simulink model "DesacopleDeTensiones"  (R2023b)
settings: Solver=VariableStepAuto  StartTime=0.0  StopTime=10.0  RelTol=1e-3
values from neighbouring files (symbols this model uses):
  L_d = 6.6 * 10^(-3)    (= 0.0066)    [varLC.m]
  L_q = 5.8 * 10^(-3)    (= 0.0058)    [varLC.m]
  lambda_m = 0.016    [varLC.m]
  P_p = 3    [Controlador.m]    (also in varLC.m)
settings Model: Creator=tomas  LastModifiedBy=gonza

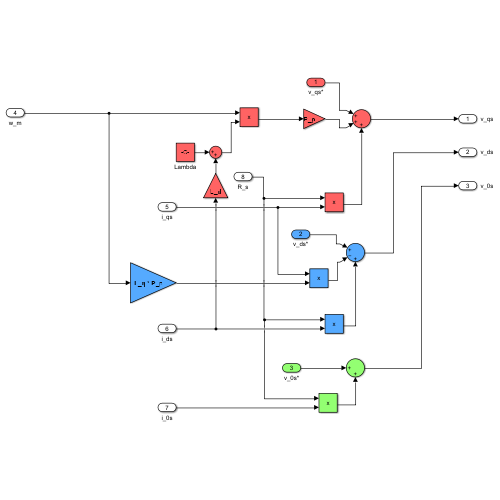
[thumbnail: Simulink's stored preview of the top-level diagram]
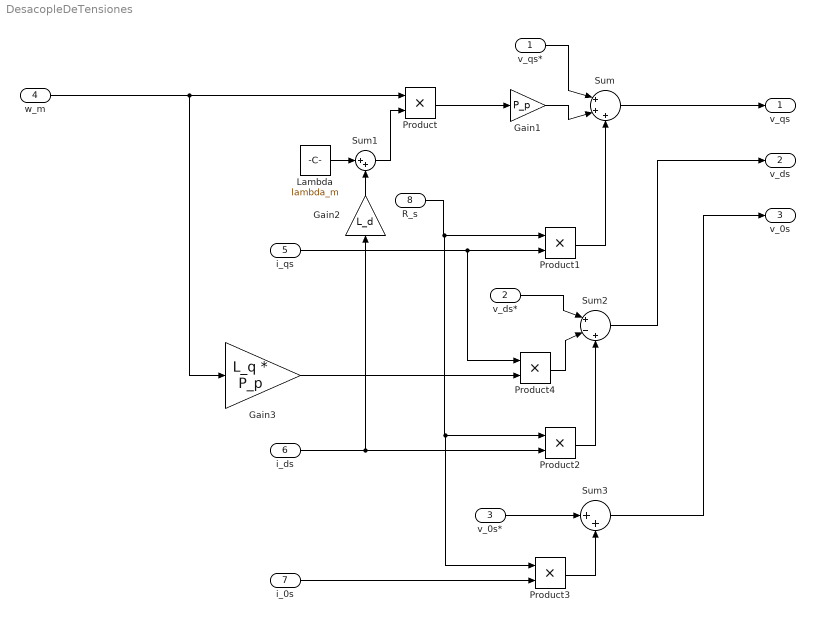
== system DesacopleDeTensiones ==
  v_qs* : Inport
  v_ds* : Inport  Port=2
  v_0s* : Inport  Port=3
  w_m : Inport  Port=4
  i_qs : Inport  Port=5
  i_ds : Inport  Port=6
  i_0s : Inport  Port=7
  R_s : Inport  Port=8
  Gain1 : Gain  Gain=P_p
  Gain2 : Gain  Gain=L_d
  Gain3 : Gain  Gain=L_q * P_p
  Lambda : Constant  Value=lambda_m
  Product{,1..4} (5 alike) : Product
  Sum : Sum  Inputs=|+++
  Sum1 : Sum  Inputs=|++
  Sum2 : Sum  Inputs=|+-+
  Sum3 : Sum  Inputs=|++
  v_qs : Outport
  v_ds : Outport  Port=2
  v_0s : Outport  Port=3
  wires:
  i_ds/1 -> Product2/2, Gain2/1
  i_qs/1 -> Product4/1, Product1/2
  Product1/1 -> Sum/3
  Gain1/1 -> Sum/2
  w_m/1 -> Gain3/1, Product/1
  Lambda/1 -> Sum1/1
  Gain2/1 -> Sum1/2
  Sum1/1 -> Product/2
  Product/1 -> Gain1/1
  v_qs*/1 -> Sum/1
  Sum/1 -> v_qs/1
  Product2/1 -> Sum2/3
  v_ds*/1 -> Sum2/1
  v_0s*/1 -> Sum3/1
  Product3/1 -> Sum3/2
  i_0s/1 -> Product3/2
  Sum3/1 -> v_0s/1
  Sum2/1 -> v_ds/1
  R_s/1 -> Product3/1, Product2/1, Product1/1
  Product4/1 -> Sum2/2
  Gain3/1 -> Product4/2
